simulink model "final_heart_sym3_3_Level_fixed"  (R2021a)
settings: Solver=VariableStepAuto  StartTime=0.0  StopTime=8  RelTol=1e-3
undefined symbols (not defined in the file or in its folder): lambda2
libraries: dspsigops x1, dspquant2 x1
(part 2 of 2)

== system final_heart_sym3_3_Level_fixed/1st_Level_Recon2/LoR_Even ==
  In_LoR_e : Inport  OutDataTypeStr=double  SampleTime=1/44100
  Add : Sum  AccumDataTypeStr=double  OutDataTypeStr=double
  Add1 : Sum  AccumDataTypeStr=double  OutDataTypeStr=double
  Delay{,1..3} (4 alike) : Delay  DelayLength=1  SampleTime=1/44100
  LoR_0 : Constant  Value=0.332670553  OutDataTypeStr=double  SampleTime=1/44100
  LoR_2 : Constant  Value=0.459877502  OutDataTypeStr=double  SampleTime=1/44100
  LoR_4 : Constant  Value=-0.085441274  OutDataTypeStr=double  SampleTime=1/44100
  Multiply : Product  OutDataTypeStr=double
  Multiply1 : Product  OutDataTypeStr=double
  Multiply2 : Product  OutDataTypeStr=double
  Rate Transition : RateTransition
  Rate Transition1 : RateTransition
  Out_LoR_e : Outport  OutDataTypeStr=double  SampleTime=1/44100  VectorParamsAs1DForOutWhenUnconnected=off
  wires:
  Delay/1 -> Rate Transition/1
  Rate Transition1/1 -> Multiply2/2
  Delay2/1 -> Add1/2
  LoR_0/1 -> Multiply/1
  Add/1 -> Out_LoR_e/1
  Delay1/1 -> Rate Transition1/1
  LoR_2/1 -> Multiply1/1
  Multiply1/1 -> Add1/1
  Rate Transition/1 -> Delay1/1, Multiply1/2
  Add1/1 -> Delay3/1
  Multiply/1 -> Add/1
  In_LoR_e/1 -> Delay/1, Multiply/2
  Multiply2/1 -> Delay2/1
  LoR_4/1 -> Multiply2/1
  Delay3/1 -> Add/2

== system final_heart_sym3_3_Level_fixed/1st_Level_Recon2/LoR_Odd ==
  In_LoR_o : Inport  OutDataTypeStr=double  SampleTime=1/44100
  Add : Sum  AccumDataTypeStr=double  OutDataTypeStr=double
  Add1 : Sum  AccumDataTypeStr=double  OutDataTypeStr=double
  Delay{,1..3} (4 alike) : Delay  DelayLength=1  SampleTime=1/44100
  LoR_1 : Constant  Value=0.806891509  OutDataTypeStr=double  SampleTime=1/44100
  LoR_3 : Constant  Value=-0.13501102  OutDataTypeStr=double  SampleTime=1/44100
  LoR_5 : Constant  Value=0.035226292  OutDataTypeStr=double  SampleTime=1/44100
  Multiply : Product  OutDataTypeStr=double
  Multiply1 : Product  OutDataTypeStr=double
  Multiply2 : Product  OutDataTypeStr=double
  Rate Transition : RateTransition
  Rate Transition1 : RateTransition
  Out_LoR_o : Outport  OutDataTypeStr=double  SampleTime=1/44100  VectorParamsAs1DForOutWhenUnconnected=off
  wires:
  Delay/1 -> Rate Transition/1
  Rate Transition1/1 -> Multiply2/2
  Delay2/1 -> Add1/2
  LoR_1/1 -> Multiply/1
  Add/1 -> Out_LoR_o/1
  Delay1/1 -> Rate Transition1/1
  LoR_3/1 -> Multiply1/1
  Multiply1/1 -> Add1/1
  Rate Transition/1 -> Delay1/1, Multiply1/2
  Add1/1 -> Delay3/1
  Multiply/1 -> Add/1
  In_LoR_o/1 -> Delay/1, Multiply/2
  Multiply2/1 -> Delay2/1
  LoR_5/1 -> Multiply2/1
  Delay3/1 -> Add/2

== system final_heart_sym3_3_Level_fixed/Heart Sound with Noise/Quantizer ==
  In1 : Inport  LockScale=on
  DTC_input_1 : DataTypeConversion  OutDataTypeStr=fixdt('double')  RndMeth=Nearest  LockScale=on
  DTC_output_1 : DataTypeConversion  OutDataTypeStr=fixdt('double')
  ReplicaOfSource : Quantizer  QuantizationInterval=0.1
  Out1 : Outport  LockScale=on
  wires:
  In1/1 -> DTC_input_1/1
  DTC_output_1/1 -> Out1/1
  ReplicaOfSource/1 -> DTC_output_1/1
  DTC_input_1/1 -> ReplicaOfSource/1

== system final_heart_sym3_3_Level_fixed/Heart Sound with Noise/Uniform Encoder ==
  In1 : Inport  LockScale=on
  DTC_input_1 : DataTypeConversion  OutDataTypeStr=fixdt('double')  RndMeth=Nearest  LockScale=on
  DTC_output_1 : DataTypeConversion  OutDataTypeStr=fixdt(0,8,0)
  ReplicaOfSource : dspquant2/Uniform Encoder  peak=2  bits=8  otype=Unsigned integer
  Out1 : Outport  LockScale=on
  wires:
  In1/1 -> DTC_input_1/1
  DTC_input_1/1 -> ReplicaOfSource/1
  DTC_output_1/1 -> Out1/1
  ReplicaOfSource/1 -> DTC_output_1/1

== system final_heart_sym3_3_Level_fixed/Threshold_Estimator/Absolute_Value1 ==
  Signal_w4 : Inport  OutDataTypeStr=double  SampleTime=1/44100
  Absolute_Switch : Switch  Threshold=1  OutDataTypeStr=double
  Constant295 : Constant  Value=0  OutDataTypeStr=double  SampleTime=1/44100
  Gain2 : Gain  Gain=-1  ParamDataTypeStr=double  OutDataTypeStr=double
  Relational Operator2 : RelationalOperator  Operator=<  OutDataTypeStr=boolean  RndMeth=Simplest
  Out_Abs : Outport  OutDataTypeStr=double  SampleTime=1/44100  VectorParamsAs1DForOutWhenUnconnected=off
  wires:
  Absolute_Switch/1 -> Out_Abs/1
  Relational Operator2/1 -> Absolute_Switch/2
  Gain2/1 -> Absolute_Switch/1
  Signal_w4/1 -> Absolute_Switch/3, Relational Operator2/1, Gain2/1
  Constant295/1 -> Relational Operator2/2

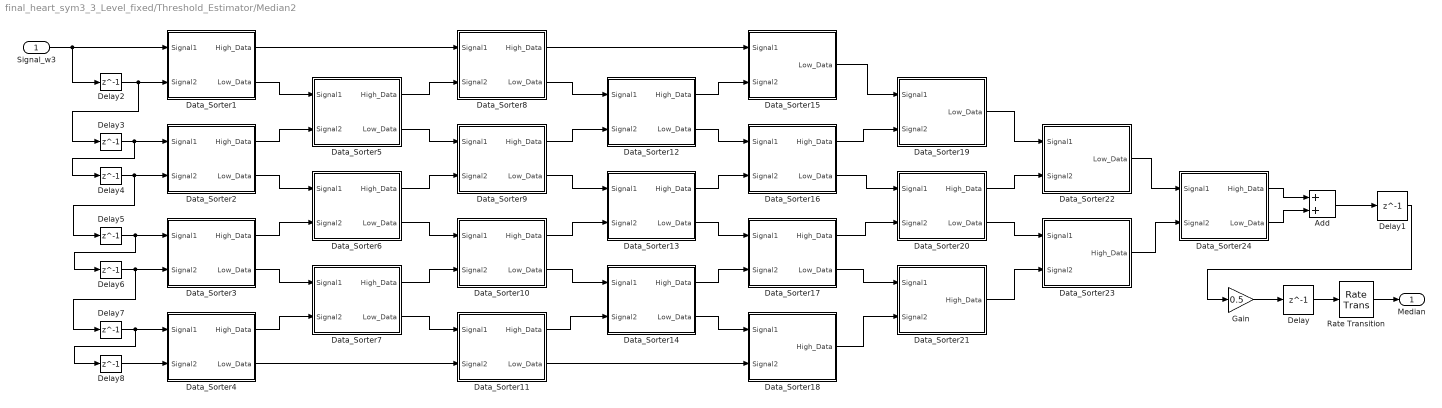
== system final_heart_sym3_3_Level_fixed/Threshold_Estimator/Median2 ==
  Signal_w3 : Inport  OutDataTypeStr=double  SampleTime=1/44100
  Add : Sum  AccumDataTypeStr=double  OutDataTypeStr=double
  Data_Sorter1 : Subsystem
  Data_Sorter10 : Subsystem
  Data_Sorter11 : Subsystem
  Data_Sorter12 : Subsystem
  Data_Sorter13 : Subsystem
  Data_Sorter14 : Subsystem
  Data_Sorter15 : Subsystem
  Data_Sorter16 : Subsystem
  Data_Sorter17 : Subsystem
  Data_Sorter18 : Subsystem
  Data_Sorter19 : Subsystem
  Data_Sorter2 : Subsystem
  Data_Sorter20 : Subsystem
  Data_Sorter21 : Subsystem
  Data_Sorter22 : Subsystem
  Data_Sorter23 : Subsystem
  Data_Sorter24 : Subsystem
  Data_Sorter3 : Subsystem
  Data_Sorter4 : Subsystem
  Data_Sorter5 : Subsystem
  Data_Sorter6 : Subsystem
  Data_Sorter7 : Subsystem
  Data_Sorter8 : Subsystem
  Data_Sorter9 : Subsystem
  Delay{,1..8} (9 alike) : Delay  DelayLength=1  SampleTime=1/44100
  Gain : Gain  Gain=0.5  ParamDataTypeStr=double  OutDataTypeStr=double
  Rate Transition : RateTransition
  Median : Outport  OutDataTypeStr=double  SampleTime=1/44100  VectorParamsAs1DForOutWhenUnconnected=off
  wires:
  Data_Sorter4/1(High_Data) -> Data_Sorter7/2(Signal2)
  Delay3/1 -> Data_Sorter2/1(Signal1), Delay4/1
  Signal_w3/1 -> Data_Sorter1/1(Signal1), Delay2/1
  Data_Sorter10/1(High_Data) -> Data_Sorter13/2(Signal2)
  Data_Sorter23/1(High_Data) -> Data_Sorter24/2(Signal2)
  Data_Sorter12/2(Low_Data) -> Data_Sorter16/1(Signal1)
  Delay2/1 -> Delay3/1, Data_Sorter1/2(Signal2)
  Data_Sorter5/1(High_Data) -> Data_Sorter8/2(Signal2)
  Delay/1 -> Rate Transition/1
  Data_Sorter15/1(Low_Data) -> Data_Sorter19/1(Signal1)
  Add/1 -> Delay1/1
  Data_Sorter7/2(Low_Data) -> Data_Sorter11/1(Signal1)
  Data_Sorter24/1(High_Data) -> Add/1
  Data_Sorter1/2(Low_Data) -> Data_Sorter5/1(Signal1)
  Data_Sorter3/1(High_Data) -> Data_Sorter6/2(Signal2)
  Data_Sorter22/1(Low_Data) -> Data_Sorter24/1(Signal1)
  Data_Sorter2/1(High_Data) -> Data_Sorter5/2(Signal2)
  Data_Sorter10/2(Low_Data) -> Data_Sorter14/1(Signal1)
  Delay1/1 -> Gain/1
  Data_Sorter17/2(Low_Data) -> Data_Sorter21/1(Signal1)
  Data_Sorter21/1(High_Data) -> Data_Sorter23/2(Signal2)
  Data_Sorter7/1(High_Data) -> Data_Sorter10/2(Signal2)
  Delay4/1 -> Data_Sorter2/2(Signal2), Delay5/1
  Data_Sorter16/1(High_Data) -> Data_Sorter19/2(Signal2)
  Data_Sorter20/1(High_Data) -> Data_Sorter22/2(Signal2)
  Data_Sorter16/2(Low_Data) -> Data_Sorter20/1(Signal1)
  Data_Sorter3/2(Low_Data) -> Data_Sorter7/1(Signal1)
  Data_Sorter2/2(Low_Data) -> Data_Sorter6/1(Signal1)
  Data_Sorter6/2(Low_Data) -> Data_Sorter10/1(Signal1)
  Data_Sorter19/1(Low_Data) -> Data_Sorter22/1(Signal1)
  Data_Sorter12/1(High_Data) -> Data_Sorter15/2(Signal2)
  Data_Sorter5/2(Low_Data) -> Data_Sorter9/1(Signal1)
  Data_Sorter24/2(Low_Data) -> Add/2
  Data_Sorter17/1(High_Data) -> Data_Sorter20/2(Signal2)
  Data_Sorter13/1(High_Data) -> Data_Sorter16/2(Signal2)
  Data_Sorter11/1(High_Data) -> Data_Sorter14/2(Signal2)
  Delay8/1 -> Data_Sorter4/2(Signal2)
  Data_Sorter8/2(Low_Data) -> Data_Sorter12/1(Signal1)
  Delay6/1 -> Data_Sorter3/2(Signal2), Delay7/1
  Data_Sorter9/2(Low_Data) -> Data_Sorter13/1(Signal1)
  Data_Sorter4/2(Low_Data) -> Data_Sorter11/2(Signal2)
  Data_Sorter9/1(High_Data) -> Data_Sorter12/2(Signal2)
  Data_Sorter14/2(Low_Data) -> Data_Sorter18/1(Signal1)
  Delay5/1 -> Data_Sorter3/1(Signal1), Delay6/1
  Delay7/1 -> Data_Sorter4/1(Signal1), Delay8/1
  Data_Sorter1/1(High_Data) -> Data_Sorter8/1(Signal1)
  Data_Sorter8/1(High_Data) -> Data_Sorter15/1(Signal1)
  Data_Sorter14/1(High_Data) -> Data_Sorter17/2(Signal2)
  Data_Sorter6/1(High_Data) -> Data_Sorter9/2(Signal2)
  Data_Sorter20/2(Low_Data) -> Data_Sorter23/1(Signal1)
  Data_Sorter11/2(Low_Data) -> Data_Sorter18/2(Signal2)
  Data_Sorter13/2(Low_Data) -> Data_Sorter17/1(Signal1)
  Gain/1 -> Delay/1
  Data_Sorter18/1(High_Data) -> Data_Sorter21/2(Signal2)
  Rate Transition/1 -> Median/1

== system final_heart_sym3_3_Level_fixed/Threshold_Estimator/Median2/Data_Sorter1 ==
  Signal1 : Inport  OutDataTypeStr=double  SampleTime=1/44100
  Signal2 : Inport  Port=2  OutDataTypeStr=double  SampleTime=1/44100
  Data_Sorter_Switch : Switch  OutDataTypeStr=double
  Data_Sorter_Switch1 : Switch  Threshold=1  OutDataTypeStr=double
  Delay1 : Delay  DelayLength=1  SampleTime=1/44100
  Delay2 : Delay  DelayLength=1  SampleTime=1/44100
  Relational Operator2 : RelationalOperator  Operator=<  OutDataTypeStr=boolean  RndMeth=Simplest
  High_Data : Outport  OutDataTypeStr=double  SampleTime=1/44100  VectorParamsAs1DForOutWhenUnconnected=off
  Low_Data : Outport  Port=2  OutDataTypeStr=double  SampleTime=1/44100  VectorParamsAs1DForOutWhenUnconnected=off
  wires:
  Signal1/1 -> Data_Sorter_Switch/3, Data_Sorter_Switch/1, Relational Operator2/1
  Relational Operator2/1 -> Data_Sorter_Switch1/2, Data_Sorter_Switch/2
  Signal2/1 -> Data_Sorter_Switch1/1, Data_Sorter_Switch1/3, Relational Operator2/2
  Data_Sorter_Switch1/1 -> Delay2/1
  Delay2/1 -> Low_Data/1
  Data_Sorter_Switch/1 -> Delay1/1
  Delay1/1 -> High_Data/1

== system final_heart_sym3_3_Level_fixed/Threshold_Estimator/Median2/Data_Sorter10 ==
  Signal1 : Inport  OutDataTypeStr=double  SampleTime=1/44100
  Signal2 : Inport  Port=2  OutDataTypeStr=double  SampleTime=1/44100
  Data_Sorter_Switch : Switch  OutDataTypeStr=double
  Data_Sorter_Switch1 : Switch  Threshold=1  OutDataTypeStr=double
  Delay1 : Delay  DelayLength=1  SampleTime=1/44100
  Delay2 : Delay  DelayLength=1  SampleTime=1/44100
  Relational Operator2 : RelationalOperator  Operator=<  OutDataTypeStr=boolean  RndMeth=Simplest
  High_Data : Outport  OutDataTypeStr=double  SampleTime=1/44100  VectorParamsAs1DForOutWhenUnconnected=off
  Low_Data : Outport  Port=2  OutDataTypeStr=double  SampleTime=1/44100  VectorParamsAs1DForOutWhenUnconnected=off
  wires:
  Signal1/1 -> Data_Sorter_Switch/3, Data_Sorter_Switch/1, Relational Operator2/1
  Relational Operator2/1 -> Data_Sorter_Switch1/2, Data_Sorter_Switch/2
  Signal2/1 -> Data_Sorter_Switch1/1, Data_Sorter_Switch1/3, Relational Operator2/2
  Data_Sorter_Switch1/1 -> Delay2/1
  Delay2/1 -> Low_Data/1
  Data_Sorter_Switch/1 -> Delay1/1
  Delay1/1 -> High_Data/1

== system final_heart_sym3_3_Level_fixed/Threshold_Estimator/Median2/Data_Sorter11 ==
  Signal1 : Inport  OutDataTypeStr=double  SampleTime=1/44100
  Signal2 : Inport  Port=2  OutDataTypeStr=double  SampleTime=1/44100
  Data_Sorter_Switch : Switch  OutDataTypeStr=double
  Data_Sorter_Switch1 : Switch  Threshold=1  OutDataTypeStr=double
  Delay1 : Delay  DelayLength=1  SampleTime=1/44100
  Delay2 : Delay  DelayLength=1  SampleTime=1/44100
  Relational Operator2 : RelationalOperator  Operator=<  OutDataTypeStr=boolean  RndMeth=Simplest
  High_Data : Outport  OutDataTypeStr=double  SampleTime=1/44100  VectorParamsAs1DForOutWhenUnconnected=off
  Low_Data : Outport  Port=2  OutDataTypeStr=double  SampleTime=1/44100  VectorParamsAs1DForOutWhenUnconnected=off
  wires:
  Signal1/1 -> Data_Sorter_Switch/3, Data_Sorter_Switch/1, Relational Operator2/1
  Relational Operator2/1 -> Data_Sorter_Switch1/2, Data_Sorter_Switch/2
  Signal2/1 -> Data_Sorter_Switch1/1, Data_Sorter_Switch1/3, Relational Operator2/2
  Data_Sorter_Switch1/1 -> Delay2/1
  Delay2/1 -> Low_Data/1
  Data_Sorter_Switch/1 -> Delay1/1
  Delay1/1 -> High_Data/1

== system final_heart_sym3_3_Level_fixed/Threshold_Estimator/Median2/Data_Sorter12 ==
  Signal1 : Inport  OutDataTypeStr=double  SampleTime=1/44100
  Signal2 : Inport  Port=2  OutDataTypeStr=double  SampleTime=1/44100
  Data_Sorter_Switch : Switch  OutDataTypeStr=double
  Data_Sorter_Switch1 : Switch  Threshold=1  OutDataTypeStr=double
  Delay1 : Delay  DelayLength=1  SampleTime=1/44100
  Delay2 : Delay  DelayLength=1  SampleTime=1/44100
  Relational Operator2 : RelationalOperator  Operator=<  OutDataTypeStr=boolean  RndMeth=Simplest
  High_Data : Outport  OutDataTypeStr=double  SampleTime=1/44100  VectorParamsAs1DForOutWhenUnconnected=off
  Low_Data : Outport  Port=2  OutDataTypeStr=double  SampleTime=1/44100  VectorParamsAs1DForOutWhenUnconnected=off
  wires:
  Signal1/1 -> Data_Sorter_Switch/3, Data_Sorter_Switch/1, Relational Operator2/1
  Relational Operator2/1 -> Data_Sorter_Switch1/2, Data_Sorter_Switch/2
  Signal2/1 -> Data_Sorter_Switch1/1, Data_Sorter_Switch1/3, Relational Operator2/2
  Data_Sorter_Switch1/1 -> Delay2/1
  Delay2/1 -> Low_Data/1
  Data_Sorter_Switch/1 -> Delay1/1
  Delay1/1 -> High_Data/1

== system final_heart_sym3_3_Level_fixed/Threshold_Estimator/Median2/Data_Sorter13 ==
  Signal1 : Inport  OutDataTypeStr=double  SampleTime=1/44100
  Signal2 : Inport  Port=2  OutDataTypeStr=double  SampleTime=1/44100
  Data_Sorter_Switch : Switch  OutDataTypeStr=double
  Data_Sorter_Switch1 : Switch  Threshold=1  OutDataTypeStr=double
  Delay1 : Delay  DelayLength=1  SampleTime=1/44100
  Delay2 : Delay  DelayLength=1  SampleTime=1/44100
  Relational Operator2 : RelationalOperator  Operator=<  OutDataTypeStr=boolean  RndMeth=Simplest
  High_Data : Outport  OutDataTypeStr=double  SampleTime=1/44100  VectorParamsAs1DForOutWhenUnconnected=off
  Low_Data : Outport  Port=2  OutDataTypeStr=double  SampleTime=1/44100  VectorParamsAs1DForOutWhenUnconnected=off
  wires:
  Signal1/1 -> Data_Sorter_Switch/3, Data_Sorter_Switch/1, Relational Operator2/1
  Relational Operator2/1 -> Data_Sorter_Switch1/2, Data_Sorter_Switch/2
  Signal2/1 -> Data_Sorter_Switch1/1, Data_Sorter_Switch1/3, Relational Operator2/2
  Data_Sorter_Switch1/1 -> Delay2/1
  Delay2/1 -> Low_Data/1
  Data_Sorter_Switch/1 -> Delay1/1
  Delay1/1 -> High_Data/1

== system final_heart_sym3_3_Level_fixed/Threshold_Estimator/Median2/Data_Sorter14 ==
  Signal1 : Inport  OutDataTypeStr=double  SampleTime=1/44100
  Signal2 : Inport  Port=2  OutDataTypeStr=double  SampleTime=1/44100
  Data_Sorter_Switch : Switch  OutDataTypeStr=double
  Data_Sorter_Switch1 : Switch  Threshold=1  OutDataTypeStr=double
  Delay1 : Delay  DelayLength=1  SampleTime=1/44100
  Delay2 : Delay  DelayLength=1  SampleTime=1/44100
  Relational Operator2 : RelationalOperator  Operator=<  OutDataTypeStr=boolean  RndMeth=Simplest
  High_Data : Outport  OutDataTypeStr=double  SampleTime=1/44100  VectorParamsAs1DForOutWhenUnconnected=off
  Low_Data : Outport  Port=2  OutDataTypeStr=double  SampleTime=1/44100  VectorParamsAs1DForOutWhenUnconnected=off
  wires:
  Signal1/1 -> Data_Sorter_Switch/3, Data_Sorter_Switch/1, Relational Operator2/1
  Relational Operator2/1 -> Data_Sorter_Switch1/2, Data_Sorter_Switch/2
  Signal2/1 -> Data_Sorter_Switch1/1, Data_Sorter_Switch1/3, Relational Operator2/2
  Data_Sorter_Switch1/1 -> Delay2/1
  Delay2/1 -> Low_Data/1
  Data_Sorter_Switch/1 -> Delay1/1
  Delay1/1 -> High_Data/1

== system final_heart_sym3_3_Level_fixed/Threshold_Estimator/Median2/Data_Sorter15 ==
  Signal1 : Inport  OutDataTypeStr=double  SampleTime=1/44100
  Signal2 : Inport  Port=2  OutDataTypeStr=double  SampleTime=1/44100
  Data_Sorter_Switch1 : Switch  Threshold=1  OutDataTypeStr=double
  Delay2 : Delay  DelayLength=1  SampleTime=1/44100
  Relational Operator2 : RelationalOperator  Operator=<  OutDataTypeStr=boolean  RndMeth=Simplest
  Low_Data : Outport  OutDataTypeStr=double  SampleTime=1/44100  VectorParamsAs1DForOutWhenUnconnected=off
  wires:
  Signal1/1 -> Relational Operator2/1
  Relational Operator2/1 -> Data_Sorter_Switch1/2
  Signal2/1 -> Data_Sorter_Switch1/1, Data_Sorter_Switch1/3, Relational Operator2/2
  Data_Sorter_Switch1/1 -> Delay2/1
  Delay2/1 -> Low_Data/1

== system final_heart_sym3_3_Level_fixed/Threshold_Estimator/Median2/Data_Sorter16 ==
  Signal1 : Inport  OutDataTypeStr=double  SampleTime=1/44100
  Signal2 : Inport  Port=2  OutDataTypeStr=double  SampleTime=1/44100
  Data_Sorter_Switch : Switch  OutDataTypeStr=double
  Data_Sorter_Switch1 : Switch  Threshold=1  OutDataTypeStr=double
  Delay1 : Delay  DelayLength=1  SampleTime=1/44100
  Delay2 : Delay  DelayLength=1  SampleTime=1/44100
  Relational Operator2 : RelationalOperator  Operator=<  OutDataTypeStr=boolean  RndMeth=Simplest
  High_Data : Outport  OutDataTypeStr=double  SampleTime=1/44100  VectorParamsAs1DForOutWhenUnconnected=off
  Low_Data : Outport  Port=2  OutDataTypeStr=double  SampleTime=1/44100  VectorParamsAs1DForOutWhenUnconnected=off
  wires:
  Signal1/1 -> Data_Sorter_Switch/3, Data_Sorter_Switch/1, Relational Operator2/1
  Relational Operator2/1 -> Data_Sorter_Switch1/2, Data_Sorter_Switch/2
  Signal2/1 -> Data_Sorter_Switch1/1, Data_Sorter_Switch1/3, Relational Operator2/2
  Data_Sorter_Switch1/1 -> Delay2/1
  Delay2/1 -> Low_Data/1
  Data_Sorter_Switch/1 -> Delay1/1
  Delay1/1 -> High_Data/1

== system final_heart_sym3_3_Level_fixed/Threshold_Estimator/Median2/Data_Sorter17 ==
  Signal1 : Inport  OutDataTypeStr=double  SampleTime=1/44100
  Signal2 : Inport  Port=2  OutDataTypeStr=double  SampleTime=1/44100
  Data_Sorter_Switch : Switch  OutDataTypeStr=double
  Data_Sorter_Switch1 : Switch  Threshold=1  OutDataTypeStr=double
  Delay1 : Delay  DelayLength=1  SampleTime=1/44100
  Delay2 : Delay  DelayLength=1  SampleTime=1/44100
  Relational Operator2 : RelationalOperator  Operator=<  OutDataTypeStr=boolean  RndMeth=Simplest
  High_Data : Outport  OutDataTypeStr=double  SampleTime=1/44100  VectorParamsAs1DForOutWhenUnconnected=off
  Low_Data : Outport  Port=2  OutDataTypeStr=double  SampleTime=1/44100  VectorParamsAs1DForOutWhenUnconnected=off
  wires:
  Signal1/1 -> Data_Sorter_Switch/3, Data_Sorter_Switch/1, Relational Operator2/1
  Relational Operator2/1 -> Data_Sorter_Switch1/2, Data_Sorter_Switch/2
  Signal2/1 -> Data_Sorter_Switch1/1, Data_Sorter_Switch1/3, Relational Operator2/2
  Data_Sorter_Switch1/1 -> Delay2/1
  Delay2/1 -> Low_Data/1
  Data_Sorter_Switch/1 -> Delay1/1
  Delay1/1 -> High_Data/1

== system final_heart_sym3_3_Level_fixed/Threshold_Estimator/Median2/Data_Sorter18 ==
  Signal1 : Inport  OutDataTypeStr=double  SampleTime=1/44100
  Signal2 : Inport  Port=2  OutDataTypeStr=double  SampleTime=1/44100
  Data_Sorter_Switch : Switch  OutDataTypeStr=double
  Delay1 : Delay  DelayLength=1  SampleTime=1/44100
  Relational Operator2 : RelationalOperator  Operator=<  OutDataTypeStr=boolean  RndMeth=Simplest
  High_Data : Outport  OutDataTypeStr=double  SampleTime=1/44100  VectorParamsAs1DForOutWhenUnconnected=off
  wires:
  Signal1/1 -> Data_Sorter_Switch/3, Data_Sorter_Switch/1, Relational Operator2/1
  Relational Operator2/1 -> Data_Sorter_Switch/2
  Signal2/1 -> Relational Operator2/2
  Data_Sorter_Switch/1 -> Delay1/1
  Delay1/1 -> High_Data/1

== system final_heart_sym3_3_Level_fixed/Threshold_Estimator/Median2/Data_Sorter19 ==
  Signal1 : Inport  OutDataTypeStr=double  SampleTime=1/44100
  Signal2 : Inport  Port=2  OutDataTypeStr=double  SampleTime=1/44100
  Data_Sorter_Switch1 : Switch  Threshold=1  OutDataTypeStr=double
  Delay2 : Delay  DelayLength=1  SampleTime=1/44100
  Relational Operator2 : RelationalOperator  Operator=<  OutDataTypeStr=boolean  RndMeth=Simplest
  Low_Data : Outport  OutDataTypeStr=double  SampleTime=1/44100  VectorParamsAs1DForOutWhenUnconnected=off
  wires:
  Signal1/1 -> Relational Operator2/1
  Relational Operator2/1 -> Data_Sorter_Switch1/2
  Signal2/1 -> Data_Sorter_Switch1/1, Data_Sorter_Switch1/3, Relational Operator2/2
  Data_Sorter_Switch1/1 -> Delay2/1
  Delay2/1 -> Low_Data/1

== system final_heart_sym3_3_Level_fixed/Threshold_Estimator/Median2/Data_Sorter2 ==
  Signal1 : Inport  OutDataTypeStr=double  SampleTime=1/44100
  Signal2 : Inport  Port=2  OutDataTypeStr=double  SampleTime=1/44100
  Data_Sorter_Switch : Switch  OutDataTypeStr=double
  Data_Sorter_Switch1 : Switch  Threshold=1  OutDataTypeStr=double
  Delay1 : Delay  DelayLength=1  SampleTime=1/44100
  Delay2 : Delay  DelayLength=1  SampleTime=1/44100
  Relational Operator2 : RelationalOperator  Operator=<  OutDataTypeStr=boolean  RndMeth=Simplest
  High_Data : Outport  OutDataTypeStr=double  SampleTime=1/44100  VectorParamsAs1DForOutWhenUnconnected=off
  Low_Data : Outport  Port=2  OutDataTypeStr=double  SampleTime=1/44100  VectorParamsAs1DForOutWhenUnconnected=off
  wires:
  Signal1/1 -> Data_Sorter_Switch/3, Data_Sorter_Switch/1, Relational Operator2/1
  Relational Operator2/1 -> Data_Sorter_Switch1/2, Data_Sorter_Switch/2
  Signal2/1 -> Data_Sorter_Switch1/1, Data_Sorter_Switch1/3, Relational Operator2/2
  Data_Sorter_Switch1/1 -> Delay2/1
  Delay2/1 -> Low_Data/1
  Data_Sorter_Switch/1 -> Delay1/1
  Delay1/1 -> High_Data/1

== system final_heart_sym3_3_Level_fixed/Threshold_Estimator/Median2/Data_Sorter20 ==
  Signal1 : Inport  OutDataTypeStr=double  SampleTime=1/44100
  Signal2 : Inport  Port=2  OutDataTypeStr=double  SampleTime=1/44100
  Data_Sorter_Switch : Switch  OutDataTypeStr=double
  Data_Sorter_Switch1 : Switch  Threshold=1  OutDataTypeStr=double
  Delay1 : Delay  DelayLength=1  SampleTime=1/44100
  Delay2 : Delay  DelayLength=1  SampleTime=1/44100
  Relational Operator2 : RelationalOperator  Operator=<  OutDataTypeStr=boolean  RndMeth=Simplest
  High_Data : Outport  OutDataTypeStr=double  SampleTime=1/44100  VectorParamsAs1DForOutWhenUnconnected=off
  Low_Data : Outport  Port=2  OutDataTypeStr=double  SampleTime=1/44100  VectorParamsAs1DForOutWhenUnconnected=off
  wires:
  Signal1/1 -> Data_Sorter_Switch/3, Data_Sorter_Switch/1, Relational Operator2/1
  Relational Operator2/1 -> Data_Sorter_Switch1/2, Data_Sorter_Switch/2
  Signal2/1 -> Data_Sorter_Switch1/1, Data_Sorter_Switch1/3, Relational Operator2/2
  Data_Sorter_Switch1/1 -> Delay2/1
  Delay2/1 -> Low_Data/1
  Data_Sorter_Switch/1 -> Delay1/1
  Delay1/1 -> High_Data/1

== system final_heart_sym3_3_Level_fixed/Threshold_Estimator/Median2/Data_Sorter21 ==
  Signal1 : Inport  OutDataTypeStr=double  SampleTime=1/44100
  Signal2 : Inport  Port=2  OutDataTypeStr=double  SampleTime=1/44100
  Data_Sorter_Switch : Switch  OutDataTypeStr=double
  Delay1 : Delay  DelayLength=1  SampleTime=1/44100
  Relational Operator2 : RelationalOperator  Operator=<  OutDataTypeStr=boolean  RndMeth=Simplest
  High_Data : Outport  OutDataTypeStr=double  SampleTime=1/44100  VectorParamsAs1DForOutWhenUnconnected=off
  wires:
  Signal1/1 -> Data_Sorter_Switch/3, Data_Sorter_Switch/1, Relational Operator2/1
  Relational Operator2/1 -> Data_Sorter_Switch/2
  Signal2/1 -> Relational Operator2/2
  Data_Sorter_Switch/1 -> Delay1/1
  Delay1/1 -> High_Data/1

== system final_heart_sym3_3_Level_fixed/Threshold_Estimator/Median2/Data_Sorter22 ==
  Signal1 : Inport  OutDataTypeStr=double  SampleTime=1/44100
  Signal2 : Inport  Port=2  OutDataTypeStr=double  SampleTime=1/44100
  Data_Sorter_Switch1 : Switch  Threshold=1  OutDataTypeStr=double
  Delay2 : Delay  DelayLength=1  SampleTime=1/44100
  Relational Operator2 : RelationalOperator  Operator=<  OutDataTypeStr=boolean  RndMeth=Simplest
  Low_Data : Outport  OutDataTypeStr=double  SampleTime=1/44100  VectorParamsAs1DForOutWhenUnconnected=off
  wires:
  Signal1/1 -> Relational Operator2/1
  Relational Operator2/1 -> Data_Sorter_Switch1/2
  Signal2/1 -> Data_Sorter_Switch1/1, Data_Sorter_Switch1/3, Relational Operator2/2
  Data_Sorter_Switch1/1 -> Delay2/1
  Delay2/1 -> Low_Data/1

== system final_heart_sym3_3_Level_fixed/Threshold_Estimator/Median2/Data_Sorter23 ==
  Signal1 : Inport  OutDataTypeStr=double  SampleTime=1/44100
  Signal2 : Inport  Port=2  OutDataTypeStr=double  SampleTime=1/44100
  Data_Sorter_Switch : Switch  OutDataTypeStr=double
  Delay1 : Delay  DelayLength=1  SampleTime=1/44100
  Relational Operator2 : RelationalOperator  Operator=<  OutDataTypeStr=boolean  RndMeth=Simplest
  High_Data : Outport  OutDataTypeStr=double  SampleTime=1/44100  VectorParamsAs1DForOutWhenUnconnected=off
  wires:
  Signal1/1 -> Data_Sorter_Switch/3, Data_Sorter_Switch/1, Relational Operator2/1
  Relational Operator2/1 -> Data_Sorter_Switch/2
  Signal2/1 -> Relational Operator2/2
  Data_Sorter_Switch/1 -> Delay1/1
  Delay1/1 -> High_Data/1

== system final_heart_sym3_3_Level_fixed/Threshold_Estimator/Median2/Data_Sorter24 ==
  Signal1 : Inport  OutDataTypeStr=double  SampleTime=1/44100
  Signal2 : Inport  Port=2  OutDataTypeStr=double  SampleTime=1/44100
  Data_Sorter_Switch : Switch  OutDataTypeStr=double
  Data_Sorter_Switch1 : Switch  Threshold=1  OutDataTypeStr=double
  Delay1 : Delay  DelayLength=1  SampleTime=1/44100
  Delay2 : Delay  DelayLength=1  SampleTime=1/44100
  Relational Operator2 : RelationalOperator  Operator=<  OutDataTypeStr=boolean  RndMeth=Simplest
  High_Data : Outport  OutDataTypeStr=double  SampleTime=1/44100  VectorParamsAs1DForOutWhenUnconnected=off
  Low_Data : Outport  Port=2  OutDataTypeStr=double  SampleTime=1/44100  VectorParamsAs1DForOutWhenUnconnected=off
  wires:
  Signal1/1 -> Data_Sorter_Switch/3, Data_Sorter_Switch/1, Relational Operator2/1
  Relational Operator2/1 -> Data_Sorter_Switch1/2, Data_Sorter_Switch/2
  Signal2/1 -> Data_Sorter_Switch1/1, Data_Sorter_Switch1/3, Relational Operator2/2
  Data_Sorter_Switch1/1 -> Delay2/1
  Delay2/1 -> Low_Data/1
  Data_Sorter_Switch/1 -> Delay1/1
  Delay1/1 -> High_Data/1

== system final_heart_sym3_3_Level_fixed/Threshold_Estimator/Median2/Data_Sorter3 ==
  Signal1 : Inport  OutDataTypeStr=double  SampleTime=1/44100
  Signal2 : Inport  Port=2  OutDataTypeStr=double  SampleTime=1/44100
  Data_Sorter_Switch : Switch  OutDataTypeStr=double
  Data_Sorter_Switch1 : Switch  Threshold=1  OutDataTypeStr=double
  Delay1 : Delay  DelayLength=1  SampleTime=1/44100
  Delay2 : Delay  DelayLength=1  SampleTime=1/44100
  Relational Operator2 : RelationalOperator  Operator=<  OutDataTypeStr=boolean  RndMeth=Simplest
  High_Data : Outport  OutDataTypeStr=double  SampleTime=1/44100  VectorParamsAs1DForOutWhenUnconnected=off
  Low_Data : Outport  Port=2  OutDataTypeStr=double  SampleTime=1/44100  VectorParamsAs1DForOutWhenUnconnected=off
  wires:
  Signal1/1 -> Data_Sorter_Switch/3, Data_Sorter_Switch/1, Relational Operator2/1
  Relational Operator2/1 -> Data_Sorter_Switch1/2, Data_Sorter_Switch/2
  Signal2/1 -> Data_Sorter_Switch1/1, Data_Sorter_Switch1/3, Relational Operator2/2
  Data_Sorter_Switch1/1 -> Delay2/1
  Delay2/1 -> Low_Data/1
  Data_Sorter_Switch/1 -> Delay1/1
  Delay1/1 -> High_Data/1

== system final_heart_sym3_3_Level_fixed/Threshold_Estimator/Median2/Data_Sorter4 ==
  Signal1 : Inport  OutDataTypeStr=double  SampleTime=1/44100
  Signal2 : Inport  Port=2  OutDataTypeStr=double  SampleTime=1/44100
  Data_Sorter_Switch : Switch  OutDataTypeStr=double
  Data_Sorter_Switch1 : Switch  Threshold=1  OutDataTypeStr=double
  Delay1 : Delay  DelayLength=1  SampleTime=1/44100
  Delay2 : Delay  DelayLength=1  SampleTime=1/44100
  Relational Operator2 : RelationalOperator  Operator=<  OutDataTypeStr=boolean  RndMeth=Simplest
  High_Data : Outport  OutDataTypeStr=double  SampleTime=1/44100  VectorParamsAs1DForOutWhenUnconnected=off
  Low_Data : Outport  Port=2  OutDataTypeStr=double  SampleTime=1/44100  VectorParamsAs1DForOutWhenUnconnected=off
  wires:
  Signal1/1 -> Data_Sorter_Switch/3, Data_Sorter_Switch/1, Relational Operator2/1
  Relational Operator2/1 -> Data_Sorter_Switch1/2, Data_Sorter_Switch/2
  Signal2/1 -> Data_Sorter_Switch1/1, Data_Sorter_Switch1/3, Relational Operator2/2
  Data_Sorter_Switch1/1 -> Delay2/1
  Delay2/1 -> Low_Data/1
  Data_Sorter_Switch/1 -> Delay1/1
  Delay1/1 -> High_Data/1

== system final_heart_sym3_3_Level_fixed/Threshold_Estimator/Median2/Data_Sorter5 ==
  Signal1 : Inport  OutDataTypeStr=double  SampleTime=1/44100
  Signal2 : Inport  Port=2  OutDataTypeStr=double  SampleTime=1/44100
  Data_Sorter_Switch : Switch  OutDataTypeStr=double
  Data_Sorter_Switch1 : Switch  Threshold=1  OutDataTypeStr=double
  Delay1 : Delay  DelayLength=1  SampleTime=1/44100
  Delay2 : Delay  DelayLength=1  SampleTime=1/44100
  Relational Operator2 : RelationalOperator  Operator=<  OutDataTypeStr=boolean  RndMeth=Simplest
  High_Data : Outport  OutDataTypeStr=double  SampleTime=1/44100  VectorParamsAs1DForOutWhenUnconnected=off
  Low_Data : Outport  Port=2  OutDataTypeStr=double  SampleTime=1/44100  VectorParamsAs1DForOutWhenUnconnected=off
  wires:
  Signal1/1 -> Data_Sorter_Switch/3, Data_Sorter_Switch/1, Relational Operator2/1
  Relational Operator2/1 -> Data_Sorter_Switch1/2, Data_Sorter_Switch/2
  Signal2/1 -> Data_Sorter_Switch1/1, Data_Sorter_Switch1/3, Relational Operator2/2
  Data_Sorter_Switch1/1 -> Delay2/1
  Delay2/1 -> Low_Data/1
  Data_Sorter_Switch/1 -> Delay1/1
  Delay1/1 -> High_Data/1

== system final_heart_sym3_3_Level_fixed/Threshold_Estimator/Median2/Data_Sorter6 ==
  Signal1 : Inport  OutDataTypeStr=double  SampleTime=1/44100
  Signal2 : Inport  Port=2  OutDataTypeStr=double  SampleTime=1/44100
  Data_Sorter_Switch : Switch  OutDataTypeStr=double
  Data_Sorter_Switch1 : Switch  Threshold=1  OutDataTypeStr=double
  Delay1 : Delay  DelayLength=1  SampleTime=1/44100
  Delay2 : Delay  DelayLength=1  SampleTime=1/44100
  Relational Operator2 : RelationalOperator  Operator=<  OutDataTypeStr=boolean  RndMeth=Simplest
  High_Data : Outport  OutDataTypeStr=double  SampleTime=1/44100  VectorParamsAs1DForOutWhenUnconnected=off
  Low_Data : Outport  Port=2  OutDataTypeStr=double  SampleTime=1/44100  VectorParamsAs1DForOutWhenUnconnected=off
  wires:
  Signal1/1 -> Data_Sorter_Switch/3, Data_Sorter_Switch/1, Relational Operator2/1
  Relational Operator2/1 -> Data_Sorter_Switch1/2, Data_Sorter_Switch/2
  Signal2/1 -> Data_Sorter_Switch1/1, Data_Sorter_Switch1/3, Relational Operator2/2
  Data_Sorter_Switch1/1 -> Delay2/1
  Delay2/1 -> Low_Data/1
  Data_Sorter_Switch/1 -> Delay1/1
  Delay1/1 -> High_Data/1

== system final_heart_sym3_3_Level_fixed/Threshold_Estimator/Median2/Data_Sorter7 ==
  Signal1 : Inport  OutDataTypeStr=double  SampleTime=1/44100
  Signal2 : Inport  Port=2  OutDataTypeStr=double  SampleTime=1/44100
  Data_Sorter_Switch : Switch  OutDataTypeStr=double
  Data_Sorter_Switch1 : Switch  Threshold=1  OutDataTypeStr=double
  Delay1 : Delay  DelayLength=1  SampleTime=1/44100
  Delay2 : Delay  DelayLength=1  SampleTime=1/44100
  Relational Operator2 : RelationalOperator  Operator=<  OutDataTypeStr=boolean  RndMeth=Simplest
  High_Data : Outport  OutDataTypeStr=double  SampleTime=1/44100  VectorParamsAs1DForOutWhenUnconnected=off
  Low_Data : Outport  Port=2  OutDataTypeStr=double  SampleTime=1/44100  VectorParamsAs1DForOutWhenUnconnected=off
  wires:
  Signal1/1 -> Data_Sorter_Switch/3, Data_Sorter_Switch/1, Relational Operator2/1
  Relational Operator2/1 -> Data_Sorter_Switch1/2, Data_Sorter_Switch/2
  Signal2/1 -> Data_Sorter_Switch1/1, Data_Sorter_Switch1/3, Relational Operator2/2
  Data_Sorter_Switch1/1 -> Delay2/1
  Delay2/1 -> Low_Data/1
  Data_Sorter_Switch/1 -> Delay1/1
  Delay1/1 -> High_Data/1

== system final_heart_sym3_3_Level_fixed/Threshold_Estimator/Median2/Data_Sorter8 ==
  Signal1 : Inport  OutDataTypeStr=double  SampleTime=1/44100
  Signal2 : Inport  Port=2  OutDataTypeStr=double  SampleTime=1/44100
  Data_Sorter_Switch : Switch  OutDataTypeStr=double
  Data_Sorter_Switch1 : Switch  Threshold=1  OutDataTypeStr=double
  Delay1 : Delay  DelayLength=1  SampleTime=1/44100
  Delay2 : Delay  DelayLength=1  SampleTime=1/44100
  Relational Operator2 : RelationalOperator  Operator=<  OutDataTypeStr=boolean  RndMeth=Simplest
  High_Data : Outport  OutDataTypeStr=double  SampleTime=1/44100  VectorParamsAs1DForOutWhenUnconnected=off
  Low_Data : Outport  Port=2  OutDataTypeStr=double  SampleTime=1/44100  VectorParamsAs1DForOutWhenUnconnected=off
  wires:
  Signal1/1 -> Data_Sorter_Switch/3, Data_Sorter_Switch/1, Relational Operator2/1
  Relational Operator2/1 -> Data_Sorter_Switch1/2, Data_Sorter_Switch/2
  Signal2/1 -> Data_Sorter_Switch1/1, Data_Sorter_Switch1/3, Relational Operator2/2
  Data_Sorter_Switch1/1 -> Delay2/1
  Delay2/1 -> Low_Data/1
  Data_Sorter_Switch/1 -> Delay1/1
  Delay1/1 -> High_Data/1

== system final_heart_sym3_3_Level_fixed/Threshold_Estimator/Median2/Data_Sorter9 ==
  Signal1 : Inport  OutDataTypeStr=double  SampleTime=1/44100
  Signal2 : Inport  Port=2  OutDataTypeStr=double  SampleTime=1/44100
  Data_Sorter_Switch : Switch  OutDataTypeStr=double
  Data_Sorter_Switch1 : Switch  Threshold=1  OutDataTypeStr=double
  Delay1 : Delay  DelayLength=1  SampleTime=1/44100
  Delay2 : Delay  DelayLength=1  SampleTime=1/44100
  Relational Operator2 : RelationalOperator  Operator=<  OutDataTypeStr=boolean  RndMeth=Simplest
  High_Data : Outport  OutDataTypeStr=double  SampleTime=1/44100  VectorParamsAs1DForOutWhenUnconnected=off
  Low_Data : Outport  Port=2  OutDataTypeStr=double  SampleTime=1/44100  VectorParamsAs1DForOutWhenUnconnected=off
  wires:
  Signal1/1 -> Data_Sorter_Switch/3, Data_Sorter_Switch/1, Relational Operator2/1
  Relational Operator2/1 -> Data_Sorter_Switch1/2, Data_Sorter_Switch/2
  Signal2/1 -> Data_Sorter_Switch1/1, Data_Sorter_Switch1/3, Relational Operator2/2
  Data_Sorter_Switch1/1 -> Delay2/1
  Delay2/1 -> Low_Data/1
  Data_Sorter_Switch/1 -> Delay1/1
  Delay1/1 -> High_Data/1
